simulink model "simCoupledStrings_R2016a"  (R2016a)
settings: Solver=VariableStepAuto  SolverMode=SingleTasking  StartTime=0.0  StopTime=20.0  RelTol=1e-3
values from neighbouring files (symbols this model uses):
  con = struct()    [fractionalCoupledSprings.m]    (also in fractionalGarrapaCoupledSprings.m; modelCoupledSprings.m; odeCoupledStrings.m; optimisation.m = eval(sprintf('con)
  par = struct()    [fractionalCoupledSprings.m]    (also in fractionalGarrapaCoupledSprings.m; modelCoupledSprings.m; odeCoupledStrings.m; optimisation.m = eval(sprintf('par)
settings Model: Creator=jkpvsz  LastModifiedBy=jkpvsz
settings DataIOCC: ReturnWorkspaceOutputs=on
settings DebuggingCC: SFUnexpectedBacktrackingDiag=error  SFNoUnconditionalDefaultTransitionDiag=error
settings SFSimCC: SimUseLocalCustomCode=on
settings RTWCC: RTWUseLocalCustomCode=on
settings GRTTargetCC: TargetLangStandard=C99 (ISO)
settings ConfigComp: CovMetricSettings=dwe  CovHtmlReporting=off  CovSaveCumulativeToWorkspaceVar=off  CovSaveSingleToWorkspaceVar=off  CovExternalEMLEnable=on

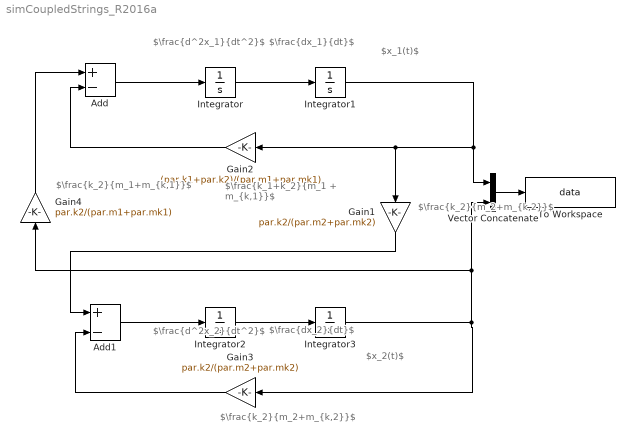
== system simCoupledStrings_R2016a ==
  note: $\frac{d^2x_1}{dt^2}$
  note: $\frac{dx_1}{dt}$
  note: $x_1(t)$
  note: $\frac{k_2}{m_2+m_{k,2}}$
  note: $\frac{k_2}{m_2+m_{k,2}}$
  note: $\frac{d^2x_2}{dt^2}$
  note: $\frac{dx_2}{dt}$
  note: $x_2(t)$
  note: $\frac{k_1+k_2}{m_1 + m_{k,1}}$
  note: $\frac{k_2}{m_1+m_{k,1}}$
  Add : Sum  Inputs=+-
  Add1 : Sum  Inputs=+-
  Gain1 : Gain  Gain=par.k2/(par.m2+par.mk2)
  Gain2 : Gain  Gain=(par.k1+par.k2)/(par.m1+par.mk1)
  Gain3 : Gain  Gain=par.k2/(par.m2+par.mk2)
  Gain4 : Gain  Gain=par.k2/(par.m1+par.mk1)
  Integrator : Integrator
  Integrator1 : Integrator  InitialCondition=con.x10
  Integrator2 : Integrator
  Integrator3 : Integrator  InitialCondition=con.x20
  To Workspace : ToWorkspace  VariableName=data  SaveFormat=Timeseries  SampleTime=-1
  Vector Concatenate : Concatenate
  wires:
  Add/1 -> Integrator/1
  Integrator/1 -> Integrator1/1
  Gain2/1 -> Add/2
  Gain3/1 -> Add1/2
  Add1/1 -> Integrator2/1
  Gain1/1 -> Add1/1
  Integrator2/1 -> Integrator3/1
  Vector Concatenate/1 -> To Workspace/1
  Gain4/1 -> Add/1
  Integrator1/1 -> Vector Concatenate/1, Gain2/1, Gain1/1
  Integrator3/1 -> Gain3/1, Vector Concatenate/2, Gain4/1
